simulink model "Loop"  (R2023b)
settings: Solver=VariableStepAuto  StartTime=0.0  StopTime=10.0  RelTol=1e-3
settings Model: Creator=jsonm  LastModifiedBy=jsonm

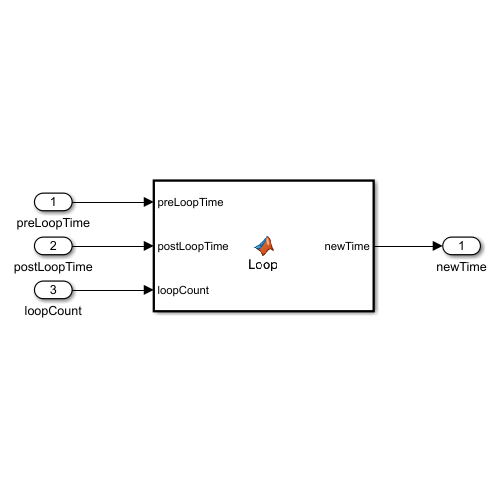
[thumbnail: Simulink's stored preview of the top-level diagram]
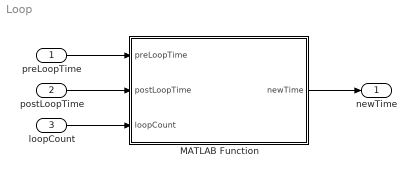
== system Loop ==
  preLoopTime : Inport
  postLoopTime : Inport  Port=2
  loopCount : Inport  Port=3
  MATLAB Function : MATLAB Function  TreatAsAtomicUnit=on
  newTime : Outport
  wires:
  preLoopTime/1 -> MATLAB Function/1(preLoopTime)
  loopCount/1 -> MATLAB Function/3(loopCount)
  postLoopTime/1 -> MATLAB Function/2(postLoopTime)
  MATLAB Function/1(newTime) -> newTime/1

== matlab function Loop/MATLAB Function ==
  data: preLoopTime input; newTime output; postLoopTime input; loopCount input
function newTime = Loop(preLoopTime, postLoopTime, loopCount)

% Function to count time generated by loops, assuming each module time has
% been estimated already.
%
% Written by: Darian Muresan

newTime = preLoopTime + loopCount*(postLoopTime - preLoopTime);
